simulink model "Power_factor_of_series_RLC_circuit"  (R2020a)
settings: Solver=VariableStepAuto  StartTime=0.0  StopTime=1  RelTol=1e-3
libraries: powerlib x7, powerlib_meascontrol x1
settings Model: Creator=ranay  LastModifiedBy=Mahsa
settings DataIOCC: ReturnWorkspaceOutputs=off
settings DebuggingCC: ArithmeticOperatorsInVariantConditions=warning
settings SFSimCC: SimUseLocalCustomCode=off  CustomCodeUndefinedFunction=UseInterfaceOnly
settings RTWCC: RTWUseLocalCustomCode=off

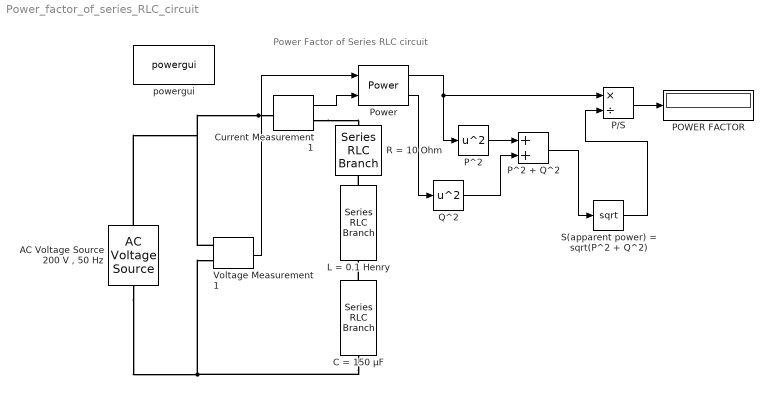
== system Power_factor_of_series_RLC_circuit ==
  note: Power Factor of Series RLC circuit
  "AC Voltage Source 200 V , 50 Hz" : powerlib/Electrical Sources/AC Voltage Source  Amplitude=200  Phase=0  Frequency=50  SampleTime=0  Measurements=None  BusType=swing  Pref=10e3  Qref=0  Qmin=-inf  Qmax=+inf
  "C = 150 µF " : powerlib/Elements/Series RLC Branch  LConnTagsString=__new0  RConnTagsString=__new0  BranchType=C  Resistance=10  Inductance=0.4  SetiL0=off  InitialCurrent=0  Capacitance=150e-6  Setx0=off  InitialVoltage=0  Measurements=None
  Current Measurement1 : powerlib/Measurements/Current Measurement  PhasorSimulation=off  OutputType=Complex  PSBequivalent=0
  L = 0.1 Henry : powerlib/Elements/Series RLC Branch  LConnTagsString=__new0  RConnTagsString=__new0  BranchType=L  Resistance=10  Inductance=0.1  SetiL0=off  InitialCurrent=0  Capacitance=1e-6  Setx0=off  InitialVoltage=0  Measurements=None
  P/S : Product  Inputs=*/
  POWER FACTOR : Display
  P^2 : Math  Operator=square  SignedPower=on  SaturateOnIntegerOverflow=on
  P^2 + Q^2 : Sum
  Power : powerlib_meascontrol/Measurements/Power  Freq=50  Vinit=[1, 0]  Iinit=[1, 0]  Ts=0
  Q^2 : Math  Operator=square  SignedPower=on  SaturateOnIntegerOverflow=on
  R = 10 Ohm : powerlib/Elements/Series RLC Branch  LConnTagsString=__new0  RConnTagsString=__new0  BranchType=R  Resistance=10  Inductance=0.4  SetiL0=off  InitialCurrent=0  Capacitance=1e-6  Setx0=off  InitialVoltage=0  Measurements=None
  S(apparent power) = sqrt(P^2 + Q^2) : Sqrt  SaturateOnIntegerOverflow=on
  Voltage Measurement1 : powerlib/Measurements/Voltage Measurement  PhasorSimulation=off  OutputType=Complex  PSBequivalent=0
  powergui : powerlib/powergui  Priority=1  SimulationMode=Discrete  SampleTime=50e-6  frequency=60  Iterations=50  frequencyindice=50  Pbase=100e6  ErrMax=1e-4  UnitsV=kV  UnitsW=MW  buscounter=0  FunctionMessages=off  echomessages=off  EnableUseOfTLC=off  CurrentSourceSwitches=off  DisableSnubberDevices=off  DisableRonSwitches=off  DisableVfSwitches=off  DisplayEquations=off  AutomaticDiscreteSolvers=off  SolverType=Tustin/Backward Euler (TBE)  Interpol=off  ExternalGateDelay=off  methode=off  Ts=100  x0status=blocks  SPID=on  SwTol=0  HookPort=off  NonlinearTolerance=1e-4  nMaxIteration=100  ContinueOnMaxIteration=off  RestoreLinks=warning  ResistiveCurrentMeasurement=off  Frange=50  Ylog=off  Xlog=off  ShowGrid=off  save=off  variable=ZData  structure=0  ZoomFFT=off  StartTime=0.0  cycles=1  DisplayStyle=1  fundamental=60  FreqAxis=off  MaxFrequency=1000  frequencyindicesteady=1  RmsSteady=1  display=off
  wires:
  Voltage Measurement1/1 -> Power/1
  Current Measurement1/1 -> Power/2
  P^2 + Q^2/1 -> S(apparent power) = sqrt(P^2 + Q^2)/1
  Q^2/1 -> P^2 + Q^2/2
  P^2/1 -> P^2 + Q^2/1
  S(apparent power) = sqrt(P^2 + Q^2)/1 -> P/S/2
  P/S/1 -> POWER FACTOR/1
  Power/2 -> Q^2/1
  Power/1 -> P^2/1, P/S/1
  connections:
  "AC Voltage Source 200 V , 50 Hz"/LConn1 -- "C = 150 µF "/RConn1 -- Voltage Measurement1/LConn2
  Current Measurement1/LConn1 -- "AC Voltage Source 200 V , 50 Hz"/RConn1 -- Voltage Measurement1/LConn1
  L = 0.1 Henry/LConn1 -- R = 10 Ohm/RConn1
  Current Measurement1/RConn1 -- R = 10 Ohm/LConn1
  "C = 150 µF "/LConn1 -- L = 0.1 Henry/RConn1
